simulink model "simulink_OBC_Diagram"  (R2025a)
settings: Solver=VariableStepAuto  StartTime=0.0  StopTime=10  RelTol=1e-3
InitFcn:
  | net = load("Retrained_Wildfire_Classification_CNN.mat");
  | imdsTest = imageDatastore("C:\Users\kiran\Documents\F.I.R.E.SAT Project\Code Files\Simulink\test", "IncludeSubfolders",true, "LabelSource","foldernames");
  | 
  | classNames = categories(imdsTest.Labels);
libraries: deeplib x1, visionsources x1, visiongeotforms x1
settings Model: Creator=kiran  LastModifiedBy=kiran

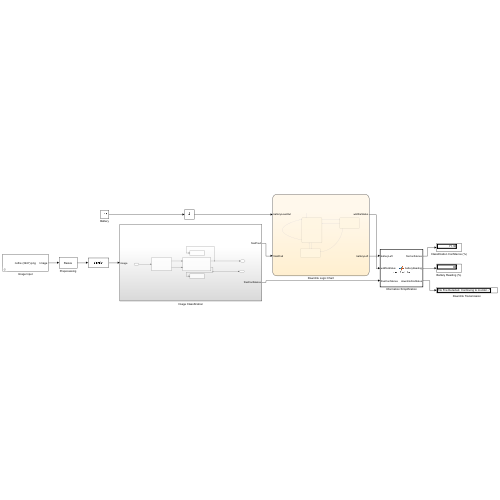
[thumbnail: Simulink's stored preview of the top-level diagram]
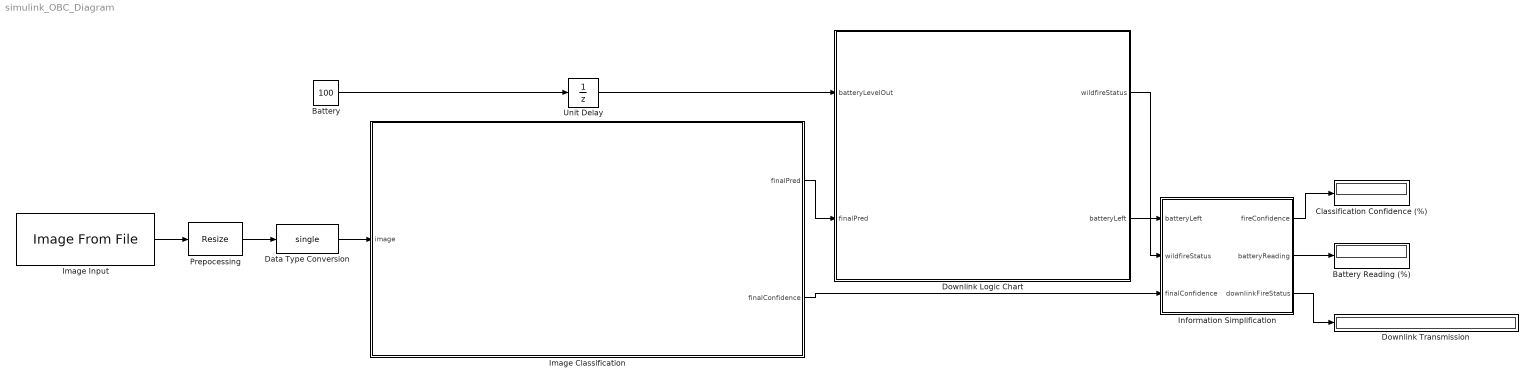
== system simulink_OBC_Diagram ==
  Battery : Constant  Value=100  OutDataTypeStr=double
  Battery Reading (%) : Display
  Classification Confidence (%) : Display
  Data Type Conversion : DataTypeConversion  OutDataTypeStr=single  SaturateOnIntegerOverflow=off  RndMeth=Floor
  Downlink Logic Chart : Stateflow chart  TreatAsAtomicUnit=on
  Downlink Transmission : Display
  Image Classification : Subsystem
  Image Input : visionsources/Image From File  Tag=vipblks_nd  FileName=C:\Users\kiran\Documents\F.I.R.E.SAT Project\Code Files\Simulink\test\nofire\nofire (3247).png  Ts=inf  imagePorts=One multidimensional signal  OutPortLabels=R|G|B  ImageDataType=uint8  sdImageDataType=uint(8)  Signed=on  WordLength=16  FractionLengthMode=User-defined  FractionLength=15
  Information Simplification : MATLAB Function  TreatAsAtomicUnit=on
  Prepocessing : visiongeotforms/Resize  specify=Output size as a percentage of input size  rfactor=[227 227]  outCols=25  outRows=25  outRowsCols=[25 35]  interp_method=Bilinear  antialias=on  useROI=off  roiFlag=off  roundingMode=Nearest  overflowMode=on  prodOutputMode=Binary point scaling  prodOutputWordLength=32  prodOutputFracLength=10
  Unit Delay : UnitDelay  InitialCondition=100  HasFrameUpgradeWarning=on
  wires:
  Image Input/1 -> Prepocessing/1
  Downlink Logic Chart/1(wildfireStatus) -> Information Simplification/2(wildfireStatus)
  Image Classification/2(finalConfidence) -> Information Simplification/3(finalConfidence)
  Unit Delay/1 -> Downlink Logic Chart/1(batteryLevelOut)
  Prepocessing/1 -> Data Type Conversion/1
  Battery/1 -> Unit Delay/1
  Image Classification/1(finalPred) -> Downlink Logic Chart/2(finalPred)
  Data Type Conversion/1 -> Image Classification/1(image)
  Downlink Logic Chart/2(batteryLeft) -> Information Simplification/1(batteryLeft)
  Information Simplification/1(fireConfidence) -> Classification Confidence (%)/1
  Information Simplification/2(batteryReading) -> Battery Reading (%)/1
  Information Simplification/3(downlinkFireStatus) -> Downlink Transmission/1

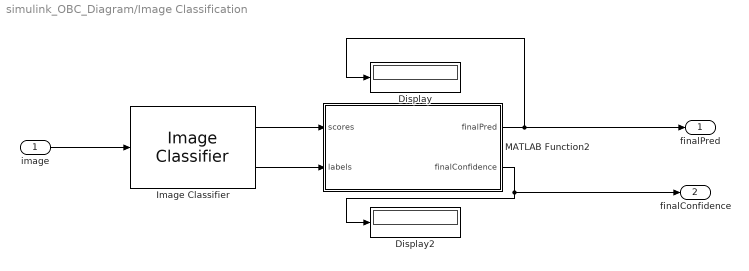
== system simulink_OBC_Diagram/Image Classification ==
  image : Inport
  Display : Display
  Display2 : Display
  Image Classifier : deeplib/Image Classifier  Network=Network from MAT-file  NetworkFunction=squeezenet  NetworkFilePath=Retrained_Wildfire_Classification_CNN.mat  NetworkClassesVariable=classNames  MiniBatchSize=128  ResizeInput=off  Classification=off  Predictions=on  ForceInterpretedSim=off  PredictMode=All probabilities and labels  K=5
  MATLAB Function2 : MATLAB Function  TreatAsAtomicUnit=on
  finalPred : Outport
  finalConfidence : Outport  Port=2
  wires:
  image/1 -> Image Classifier/1
  MATLAB Function2/2(finalConfidence) -> finalConfidence/1, Display2/1
  MATLAB Function2/1(finalPred) -> finalPred/1, Display/1
  Image Classifier/1 -> MATLAB Function2/1(scores)
  Image Classifier/2 -> MATLAB Function2/2(labels)

== matlab function simulink_OBC_Diagram/Information Simplification ==
  data: fireConfidence output; batteryReading output; downlinkFireStatus output string; batteryLeft input; wildfireStatus input; finalConfidence input
function [fireConfidence, batteryReading, downlinkFireStatus] = simplifiedInfo(batteryLeft, wildfireStatus, finalConfidence)

fireConfidence = single(0);
batteryReading = single(batteryLeft);
downlinkFireStatus = "";

if wildfireStatus == 10 && batteryLeft > 5
    fireConfidence = single(finalConfidence);
    downlinkFireStatus = "Wildfire Detected!";
elseif batteryLeft < 5
    fireConfidence = single(NaN);
    downlinkFireStatus = "Battery too low. Entering Safe Mode...";
elseif wildfireStatus == 0 && batteryLeft > 5
    fireConfidence = single(finalConfidence);
    downlinkFireStatus = "No Fire Detected. Continuing to monitor...";
end

== stateflow chart simulink_OBC_Diagram/Downlink Logic Chart ==
  state Idle
    entry:
    if finalPred == 1 || finalPred == 0
    wildfireStatus = double(finalPred);
    end
    during:
    if double(finalPred) ~= prevFinalPred
    prevFinalPred = double(finalPred);
    signal = 3;
    wildfireStatus = double(finalPred);
    end
    if signal == 3
    if finalPred == 1 && batteryLevelOut >= 5
    signal = 1;
    powerUsed = powerUsed + 4;
    elseif finalPred == 1 && batteryLevelOut < 5
    signal = 0;
    wildfireStatus = -1;
    powerUsed = powerUsed + 2;
    elseif finalPred == 0 && batteryLevelOut >= 5
    signal = 2;
    powerUsed = powerUsed + 2;
    elseif finalPred == 0 && batteryLevelOut < 5
    signal = 0;
    powerUsed = powerUsed + 2;
    end
    end
    batteryLeft = batteryLevelOut - powerUsed;
  state ReadyToTransmit
    entry:
    signal = 1;
    wildfireStatus = wildfireStatus + 1;
    during:
    if finalPred == 1 && batteryLevelOut > 5
    wildfireStatus = wildfireStatus + 1;
    elseif batteryLevelOut < 5
    wildfireStatus = -1;
    signal = 0;
    end
  state LowBattery
    entry:
    signal = 0;
    if batteryLeft < 0
    batteryLeft = 0;
    end
    during:
    batteryLeft = batteryLevelOut - powerUsed;
    end
  (default) -> Idle
  Idle -> Idle [order 3] : [signal ==2]{signal = 4;}
  Idle -> ReadyToTransmit [order 1] : [signal == 1]{signal = 4;}
  ReadyToTransmit -> Idle [order 1] : [finalPred == 0]
  ReadyToTransmit -> LowBattery [order 2] : [batteryLevelOut < 5]
  LowBattery -> Idle : [batteryLevelOut >= 15]
  Idle -> LowBattery [order 2] : [signal == 0]{signal = 4;}
  data: batteryLevelOut input; finalPred input; wildfireStatus output double; signal local double =3; powerUsed local double size=1 =0; batteryLeft output double; prevFinalPred local double =-1

== matlab function simulink_OBC_Diagram/Image Classification/MATLAB Function2 ==
  data: finalPred output; finalConfidence output; scores input; labels input
function [finalPred, finalConfidence] = predOut(scores, labels)

    finalConfidence = (max([scores(1), scores(2)])*100);
    
    if finalConfidence == scores(2)*100
        finalPred = false;
    else
        finalPred = true;
    end

end
